simulink model "SM_Tq_Ctrl"  (R2023a)
settings: Solver=ode45  StartTime=0  StopTime=20  FixedStep=0.001  RelTol=1e-3  AbsTol=1e-6
libraries: simulink x11, dspsigops x4, Solver_SF x1
settings Model: ExtModeTrigMode=oneshot  Creator=jhu  LastModifiedBy=USER
settings SolverCC: AutoScaleAbsTol=off  AlgebraicLoopSolver=TrustRegion
settings DataIOCC: SaveFormat=Array  SignalLoggingSaveFormat=ModelDataLogs  ReturnWorkspaceOutputs=off  SignalLoggingName=sigsOut
settings OptimizationCC: BlockReduction=off  BooleanDataType=off  ExpressionDepthLimit=2147483647  LifeSpan=inf
settings DebuggingCC: SaveWithParameterizedLinksMsg=none  UnderspecifiedInitializationDetection=Classic  MergeDetectMultiDrivingBlocksExec=none  SignalResolutionControl=TryResolveAllWithWarning  MultiTaskDSMMsg=warning  MultiTaskCondExecSysMsg=none  FcnCallInpInsideContextMsg=warning  UnconnectedInputMsg=warning  UnconnectedOutputMsg=warning  UnconnectedLineMsg=warning  StateNameClashWarn=warning  SFUnexpectedBacktrackingDiag=warning  SFNoUnconditionalDefaultTransitionDiag=warning  SFExecutionAtInitializationDiag=none  ArithmeticOperatorsInVariantConditions=warning
settings HardwareCC: ProdBitPerPointer=32  ProdBitPerSizeT=32  ProdBitPerPtrDiffT=32  ProdLargestAtomicFloat=None  ProdIntDivRoundTo=Undefined  ProdEndianess=Unspecified  ProdWordSize=32  ProdHWDeviceType=32-bit Generic  TargetUnknown=on
settings ModelReferenceCC: PropagateSignalLabelsOutOfModel=off
settings SFSimCC: SimUseLocalCustomCode=off  CustomCodeUndefinedFunction=UseInterfaceOnly
settings RTWCC: TemplateMakefile=grt_vc.tmf  RTWUseLocalCustomCode=off
settings CodeAppCC: StateflowObjectComments=on
settings GRTTargetCC: TargetFcnLib=ansi_tfl_tmw.mat  TargetLangStandard=C89/C90 (ANSI)  CombineOutputUpdateFcns=off  GRTInterface=on
settings ConfigComp: CovMetricSettings=dw  CovSaveCumulativeToWorkspaceVar=on  CovSaveSingleToWorkspaceVar=on  CovExternalEMLEnable=off

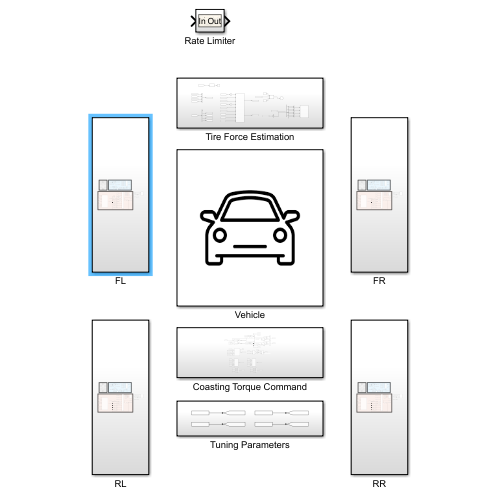
[thumbnail: Simulink's stored preview of the top-level diagram]
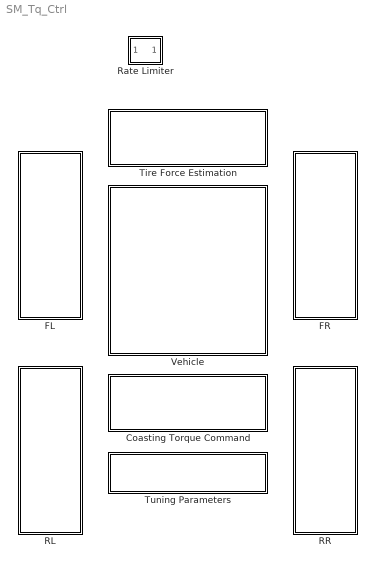
== system SM_Tq_Ctrl ==
  Coasting Torque Command : Subsystem
  FL : Subsystem
  FR : Subsystem
  RL : Subsystem
  RR : Subsystem
  Rate Limiter : Subsystem
  Tire Force Estimation : Subsystem
  Tuning Parameters : Subsystem
  Vehicle : Subsystem
      mask Display: image('C:\Users\USER\Downloads\vehicle_icon.png'); % Use "Edit Image" on toolstrip to change.

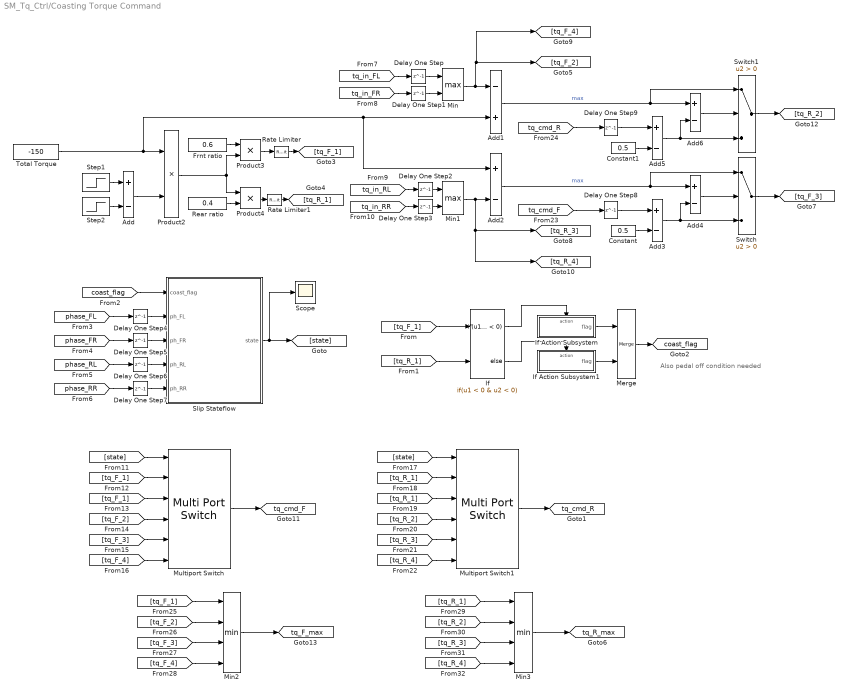
== system SM_Tq_Ctrl/Coasting Torque Command ==
  note: Also pedal off condition needed
  Add{,2..6} (6 alike) : Sum  Inputs=+-
  Add1 : Sum  Inputs=-+
  Constant : Constant  Value=0.5
  Constant1 : Constant  Value=0.5
  Delay One Step{,1..7} (8 alike) : Delay  DelayLength=1
  Delay One Step8 : Delay  DelayLength=1  SampleTime=0.01
  Delay One Step9 : Delay  DelayLength=1  SampleTime=0.01
  Frnt ratio : Constant  Value=0.6  SampleTime=0.01
  If : If  NumInputs=2  IfExpression=u1 < 0 & u2 < 0
  If Action Subsystem : Subsystem  TreatAsAtomicUnit=on
  If Action Subsystem1 : Subsystem  TreatAsAtomicUnit=on
  Merge : Merge
  Min : MinMax  Function=max  Inputs=2
  Min1 : MinMax  Function=max  Inputs=2
  Min2 : MinMax  Inputs=4
  Min3 : MinMax  Inputs=4
  Multiport Switch : MultiPortSwitch  DataPortOrder=Zero-based contiguous  Inputs=5  zeroidx=on  SaturateOnIntegerOverflow=off  InputSameDT=off
  Multiport Switch1 : MultiPortSwitch  DataPortOrder=Zero-based contiguous  Inputs=5  zeroidx=on  SaturateOnIntegerOverflow=off  InputSameDT=off
  Product2 : Product
  Product3 : Product
  Product4 : Product
  Rate Limiter : RateLimiter  RisingSlewLimit=600  FallingSlewLimit=-600  SampleTimeMode=inherited
  Rate Limiter1 : RateLimiter  RisingSlewLimit=600  FallingSlewLimit=-600  SampleTimeMode=inherited
  Rear ratio : Constant  Value=0.4  SampleTime=0.01
  Scope : Scope
  Slip Stateflow : Stateflow chart  TreatAsAtomicUnit=on
  Step1 : Step  Time=5  SampleTime=0.01
  Step2 : Step  Time=10  SampleTime=0.01
  Switch : Switch  Criteria=u2 > Threshold  SaturateOnIntegerOverflow=off  InputSameDT=off
  Switch1 : Switch  Criteria=u2 > Threshold  SaturateOnIntegerOverflow=off  InputSameDT=off
  Total Torque : Constant  Value=-150  VectorParams1D=off  SampleTime=0.01
  tag scope: coast_flag=global, tq_F_max=global, tq_R_max=global, tq_cmd_F=global, tq_cmd_R=global
  wires:
  [tq_F_1] -> If/1
  [tq_R_1] -> If/2
  If/1 -> If Action Subsystem/Action
  If Action Subsystem/1(flag) -> Merge/1
  If Action Subsystem1/1(flag) -> Merge/2
  If/2 -> If Action Subsystem1/Action
  Merge/1 -> [coast_flag]
  [coast_flag] -> Slip Stateflow/1(coast_flag)
  [phase_FL] -> Delay One Step4/1
  [phase_FR] -> Delay One Step5/1
  [phase_RL] -> Delay One Step6/1
  [phase_RR] -> Delay One Step7/1
  Slip Stateflow/1(state) -> Scope/1, [state]
  Step1/1 -> Add/1
  Step2/1 -> Add/2
  Add/1 -> Product2/2
  Product2/1 -> Product4/1, Product3/2
  Frnt ratio/1 -> Product3/1
  Rear ratio/1 -> Product4/2
  Product3/1 -> Rate Limiter/1
  Product4/1 -> Rate Limiter1/1
  [tq_in_FL] -> Delay One Step/1
  [tq_in_FR] -> Delay One Step1/1
  Min/1 -> [tq_F_4], [tq_F_2], Add1/1
  [tq_in_RL] -> Delay One Step2/1
  [tq_in_RR] -> Delay One Step3/1
  Min1/1 -> [tq_R_4], [tq_R_3], Add2/2
  Add2/1 -> Switch/1, Add4/1  "max"
  [state] -> Multiport Switch/1
  [tq_F_1] -> Multiport Switch/2
  [tq_F_1] -> Multiport Switch/3
  [tq_F_2] -> Multiport Switch/4
  [tq_F_3] -> Multiport Switch/5
  [tq_F_4] -> Multiport Switch/6
  Multiport Switch/1 -> [tq_cmd_F]
  Multiport Switch1/1 -> [tq_cmd_R]
  [tq_R_3] -> Multiport Switch1/5
  [tq_R_4] -> Multiport Switch1/6
  [tq_R_2] -> Multiport Switch1/4
  [tq_R_1] -> Multiport Switch1/2
  [state] -> Multiport Switch1/1
  [tq_R_1] -> Multiport Switch1/3
  Delay One Step/1 -> Min/1
  Delay One Step1/1 -> Min/2
  Delay One Step2/1 -> Min1/1
  Delay One Step3/1 -> Min1/2
  Delay One Step4/1 -> Slip Stateflow/2(ph_FL)
  Delay One Step5/1 -> Slip Stateflow/3(ph_FR)
  Delay One Step6/1 -> Slip Stateflow/4(ph_RL)
  Delay One Step7/1 -> Slip Stateflow/5(ph_RR)
  [tq_cmd_F] -> Delay One Step8/1
  Delay One Step8/1 -> Add3/1
  Constant/1 -> Add3/2
  Add3/1 -> Add4/2, Switch/3
  Add4/1 -> Switch/2
  Switch/1 -> [tq_F_3]
  Switch1/1 -> [tq_R_2]
  Delay One Step9/1 -> Add5/1
  Add1/1 -> Switch1/1, Add6/1  "max"
  Add6/1 -> Switch1/2
  [tq_cmd_R] -> Delay One Step9/1
  Add5/1 -> Add6/2, Switch1/3
  Constant1/1 -> Add5/2
  Min2/1 -> [tq_F_max]
  [tq_F_1] -> Min2/1
  [tq_F_2] -> Min2/2
  [tq_F_3] -> Min2/3
  [tq_F_4] -> Min2/4
  Min3/1 -> [tq_R_max]
  [tq_R_1] -> Min3/1
  [tq_R_2] -> Min3/2
  [tq_R_3] -> Min3/3
  [tq_R_4] -> Min3/4
  Total Torque/1 -> Add2/1, Add1/2, Product2/1
  Rate Limiter/1 -> [tq_F_1]
  Rate Limiter1/1 -> [tq_R_1]

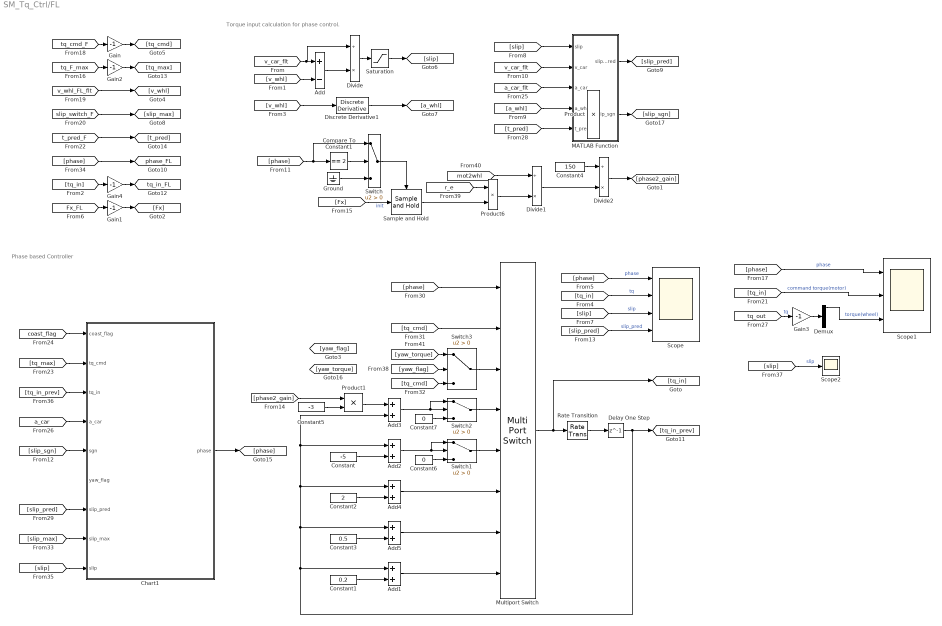
== system SM_Tq_Ctrl/FL ==
  note: Phase based Controller
  note: Torque input calculation for phase control.
  Add : Sum  Inputs=+-
  Add{1..5} (5 alike) : Sum
  Chart1 : Stateflow chart  TreatAsAtomicUnit=on
      settings: PortSchema="{\"entries\":[{\"content\":{\"sides\":[{\"content\":{\"connectorIds\":[\"In3\",\"In6\",\"In7\",\"In2\",\"In8\",\"In9\",\"In4\",\"In5\",\"In1\"]},\"type\":\"ConnectorPlacement.EquallySpacedRectSide\",\"uuid\":\"d1b40d47-5080-4bdb-9b64-2db0b8a6d570\"},{\"content\":{\"connectorIds\":[\"Out1\"],\"side\":\"RIGHT\"},\"type\":\"ConnectorPlacement.EquallySpacedRectSide\",\"uuid\":\"3562d231-244b-4945-a90c-51a654d62f0f\"},{\"content\":{\"side\":\"TOP\"},\"type\":\"ConnectorPlacement.EquallySpacedRectSide\",\"uuid\":\"6c914ffe-04dc-4ab2-bade-76d69248353c\"}]},\"type\":\"ConnectorPlacement.EquallySpacedConnector\",\"uuid\":\"36a59ec9-6bc3-461d-a020-c1da85e3b47f\"}],\"packageUris\":[\"http://schema.mathworks.com/mf0/Connector/R2020b\"],\"version\":\"1.0\"}"
  Compare To Constant1 : simulink/Logic and Bit Operations/Compare To Constant  relop===  const=2  OutDataTypeStr=boolean
  Constant : Constant  Value=-5
  Constant1 : Constant  Value=0.2
  Constant2 : Constant  Value=2
  Constant3 : Constant  Value=0.5
  Constant4 : Constant  Value=150
  Constant5 : Constant  Value=-3
  Constant6 : Constant  Value=0
  Constant7 : Constant  Value=0
  Delay One Step : Delay  DelayLength=1  SampleTime=0.01
  Demux : Demux
  Discrete Derivative1 : simulink/Discrete/Discrete Derivative  gainval=1.0  ICPrevScaledInput=0.0  OutMin=[]  OutMax=[]  OutDataType=fixdt(1, 16)  OutScaling=2^-10  DoSatur=off
  Divide : Product  Inputs=/*
  Divide1 : Product  Inputs=/*
  Divide2 : Product  Inputs=/*
  Gain{,1..4} (5 alike) : Gain  Gain=-1
  Ground : Ground
  MATLAB Function : MATLAB Function  TreatAsAtomicUnit=on
  Multiport Switch : MultiPortSwitch  DataPortOrder=Zero-based contiguous  Inputs=7  zeroidx=on  SaturateOnIntegerOverflow=off  InputSameDT=off
  Product : Product
  Product1 : Product
  Product6 : Product
  Rate Transition : RateTransition  OutPortSampleTime=0.01
  Sample and Hold : dspsigops/Sample and Hold  trig=Rising edge  initCond=0  latchinput=off
  Saturation : Saturate  UpperLimit=1  LowerLimit=-1
  Scope : Scope  NumInputPorts=4
  Scope1 : Scope  NumInputPorts=3
  Scope2 : Scope
  Switch{,1..3} (4 alike) : Switch  Criteria=u2 > Threshold  SaturateOnIntegerOverflow=off  InputSameDT=off
  tag scope: phase_FL=global, tq_in_FL=global
  wires:
  [v_car_flt] -> Divide/1, Add/1
  [v_whl] -> Add/2
  Add/1 -> Divide/2
  Divide/1 -> Saturation/1
  Saturation/1 -> [slip]
  [v_whl] -> Discrete Derivative1/1
  Discrete Derivative1/1 -> [a_whl]
  [slip_switch_F] -> [slip_max]
  [v_whl_FL_flt] -> [v_whl]
  [phase] -> Multiport Switch/1
  [tq_cmd] -> Multiport Switch/2
  [tq_cmd] -> Switch3/3
  Rate Transition/1 -> Delay One Step/1
  [slip] -> MATLAB Function/1(slip)
  [a_whl] -> MATLAB Function/4(a_whl)
  [v_car_flt] -> MATLAB Function/2(v_car)
  MATLAB Function/1(slip_pred) -> [slip_pred]
  [t_pred_F] -> [t_pred]
  [t_pred] -> MATLAB Function/5(t_pred)
  Add2/1 -> Switch1/1, Switch1/2
  Gain/1 -> [tq_cmd]
  Multiport Switch/1 -> [tq_in], Rate Transition/1
  Add4/1 -> Multiport Switch/6
  Constant2/1 -> Add4/2
  Constant3/1 -> Add5/2
  Add5/1 -> Multiport Switch/7
  Ground/1 -> Switch/3
  Switch/1 -> Sample and Hold/Trigger
  Sample and Hold/1 -> Product6/2
  [phase] -> Switch/1, Compare To Constant1/1
  Compare To Constant1/1 -> Switch/2
  Delay One Step/1 -> [tq_in_prev], Add3/2, Add2/1, Add4/1, Add5/1, Add1/1
  [Fx] -> Sample and Hold/1  "init"
  [tq_max] -> Chart1/6(tq_cmd)
  [coast_flag] -> Chart1/3(coast_flag)
  Chart1/1(phase) -> [phase]
  [a_car] -> Chart1/2(a_car)
  [slip_sgn] -> Chart1/8(sgn)
  [slip_pred] -> Chart1/4(slip_pred)
  [slip_max] -> Chart1/5(slip_max)
  [slip] -> Chart1/1(slip)
  [tq_in_prev] -> Chart1/7(tq_in)
  [phase] -> Scope/1  "phase"
  [tq_in] -> Scope/2  "tq"
  [slip] -> Scope/3  "slip"
  Divide1/1 -> Divide2/2
  [slip_pred] -> Scope/4  "slip_pred"
  Add3/1 -> Switch2/1, Switch2/2
  [phase] -> [phase_FL]
  [tq_cmd_F] -> Gain/1
  [tq_F_max] -> Gain2/1
  Gain2/1 -> [tq_max]
  [a_car_flt] -> MATLAB Function/3(a_car)
  [tq_in] -> Gain4/1
  Gain4/1 -> [tq_in_FL]
  [Fx_FL] -> Gain1/1
  Gain1/1 -> [Fx]
  [r_e] -> Product6/1
  Product6/1 -> Divide1/2
  [mot2whl] -> Divide1/1
  Constant/1 -> Add2/2
  Add1/1 -> Multiport Switch/8
  Constant1/1 -> Add1/2
  MATLAB Function/2(slip_sgn) -> [slip_sgn]
  [phase] -> Scope1/1  "phase"
  [tq_in] -> Scope1/2  "command torque(motor)"
  [tq_out] -> Gain3/1  "tq"
  Gain3/1 -> Demux/1
  Demux/1 -> Scope1/3  "torque(wheel)"
  [slip] -> Scope2/1  "slip"
  Divide2/1 -> [phase2_gain]
  Constant4/1 -> Divide2/1
  [phase2_gain] -> Product1/1
  Constant5/1 -> Product1/2
  Product1/1 -> Add3/1
  Switch1/1 -> Multiport Switch/5
  Constant6/1 -> Switch1/3
  Switch2/1 -> Multiport Switch/4
  Constant7/1 -> Switch2/3
  [yaw_flag] -> Switch3/2
  [yaw_torque] -> Switch3/1
  Switch3/1 -> Multiport Switch/3

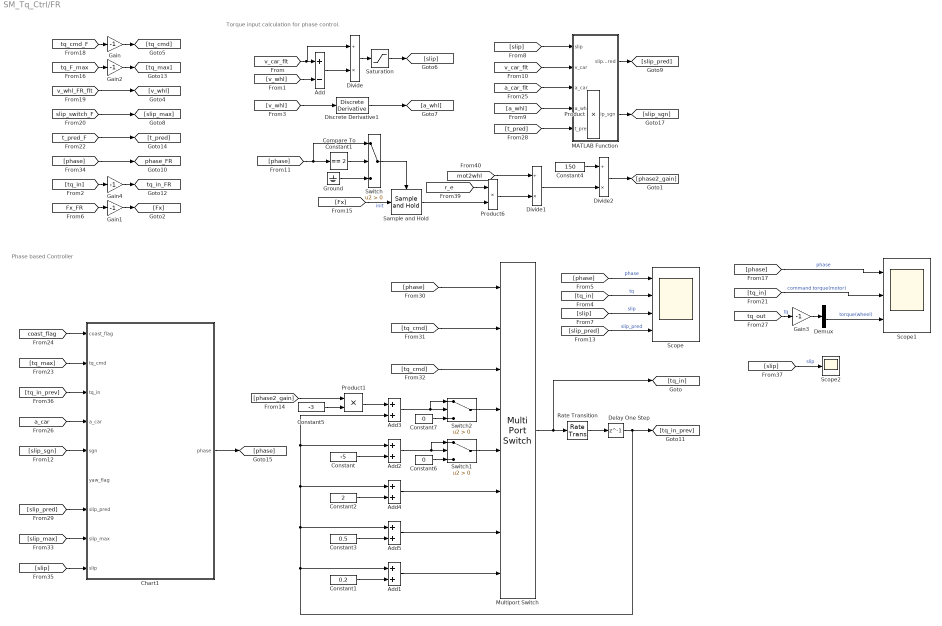
== system SM_Tq_Ctrl/FR ==
  note: Torque input calculation for phase control.
  note: Phase based Controller
  Add : Sum  Inputs=+-
  Add{1..5} (5 alike) : Sum
  Chart1 : Stateflow chart  TreatAsAtomicUnit=on
      settings: PortSchema="{\"entries\":[{\"content\":{\"sides\":[{\"content\":{\"connectorIds\":[\"In3\",\"In6\",\"In7\",\"In2\",\"In8\",\"In9\",\"In4\",\"In5\",\"In1\"]},\"type\":\"ConnectorPlacement.EquallySpacedRectSide\",\"uuid\":\"d1b40d47-5080-4bdb-9b64-2db0b8a6d570\"},{\"content\":{\"connectorIds\":[\"Out1\"],\"side\":\"RIGHT\"},\"type\":\"ConnectorPlacement.EquallySpacedRectSide\",\"uuid\":\"3562d231-244b-4945-a90c-51a654d62f0f\"},{\"content\":{\"side\":\"TOP\"},\"type\":\"ConnectorPlacement.EquallySpacedRectSide\",\"uuid\":\"6c914ffe-04dc-4ab2-bade-76d69248353c\"}]},\"type\":\"ConnectorPlacement.EquallySpacedConnector\",\"uuid\":\"36a59ec9-6bc3-461d-a020-c1da85e3b47f\"}],\"packageUris\":[\"http://schema.mathworks.com/mf0/Connector/R2020b\"],\"version\":\"1.0\"}"
  Compare To Constant1 : simulink/Logic and Bit Operations/Compare To Constant  relop===  const=2  OutDataTypeStr=boolean
  Constant : Constant  Value=-5
  Constant1 : Constant  Value=0.2
  Constant2 : Constant  Value=2
  Constant3 : Constant  Value=0.5
  Constant4 : Constant  Value=150
  Constant5 : Constant  Value=-3
  Constant6 : Constant  Value=0
  Constant7 : Constant  Value=0
  Delay One Step : Delay  DelayLength=1  SampleTime=0.01
  Demux : Demux
  Discrete Derivative1 : simulink/Discrete/Discrete Derivative  gainval=1.0  ICPrevScaledInput=0.0  OutMin=[]  OutMax=[]  OutDataType=fixdt(1, 16)  OutScaling=2^-10  DoSatur=off
  Divide : Product  Inputs=/*
  Divide1 : Product  Inputs=/*
  Divide2 : Product  Inputs=/*
  Gain{,1..4} (5 alike) : Gain  Gain=-1
  Ground : Ground
  MATLAB Function : MATLAB Function  TreatAsAtomicUnit=on
  Multiport Switch : MultiPortSwitch  DataPortOrder=Zero-based contiguous  Inputs=7  zeroidx=on  SaturateOnIntegerOverflow=off  InputSameDT=off
  Product : Product
  Product1 : Product
  Product6 : Product
  Rate Transition : RateTransition  OutPortSampleTime=0.01
  Sample and Hold : dspsigops/Sample and Hold  trig=Rising edge  initCond=0  latchinput=off
  Saturation : Saturate  UpperLimit=1  LowerLimit=-1
  Scope : Scope  NumInputPorts=4
  Scope1 : Scope  NumInputPorts=3
  Scope2 : Scope
  Switch : Switch  Criteria=u2 > Threshold  SaturateOnIntegerOverflow=off  InputSameDT=off
  Switch1 : Switch  Criteria=u2 > Threshold  SaturateOnIntegerOverflow=off  InputSameDT=off
  Switch2 : Switch  Criteria=u2 > Threshold  SaturateOnIntegerOverflow=off  InputSameDT=off
  tag scope: phase_FR=global, tq_in_FR=global
  wires:
  Constant7/1 -> Switch2/3
  Switch2/1 -> Multiport Switch/4
  Constant6/1 -> Switch1/3
  Switch1/1 -> Multiport Switch/5
  Product1/1 -> Add3/1
  Constant5/1 -> Product1/2
  [phase2_gain] -> Product1/1
  Constant4/1 -> Divide2/1
  Divide2/1 -> [phase2_gain]
  [slip] -> Scope2/1  "slip"
  Demux/3 -> Scope1/3  "torque(wheel)"
  Gain3/1 -> Demux/1
  [tq_out] -> Gain3/1  "tq"
  [tq_in] -> Scope1/2  "command torque(motor)"
  [phase] -> Scope1/1  "phase"
  MATLAB Function/2(slip_sgn) -> [slip_sgn]
  Constant1/1 -> Add1/2
  Add1/1 -> Multiport Switch/8
  Constant/1 -> Add2/2
  [mot2whl] -> Divide1/1
  Product6/1 -> Divide1/2
  [r_e] -> Product6/1
  Gain1/1 -> [Fx]
  [Fx_FR] -> Gain1/1
  Gain4/1 -> [tq_in_FR]
  [tq_in] -> Gain4/1
  [a_car_flt] -> MATLAB Function/3(a_car)
  Gain2/1 -> [tq_max]
  [tq_F_max] -> Gain2/1
  [tq_cmd_F] -> Gain/1
  [phase] -> [phase_FR]
  Add3/1 -> Switch2/2, Switch2/1
  [slip_pred] -> Scope/4  "slip_pred"
  Divide1/1 -> Divide2/2
  [slip] -> Scope/3  "slip"
  [tq_in] -> Scope/2  "tq"
  [phase] -> Scope/1  "phase"
  [tq_in_prev] -> Chart1/7(tq_in)
  [slip] -> Chart1/1(slip)
  [slip_max] -> Chart1/5(slip_max)
  [slip_pred] -> Chart1/4(slip_pred)
  [slip_sgn] -> Chart1/8(sgn)
  [a_car] -> Chart1/2(a_car)
  Chart1/1(phase) -> [phase]
  [coast_flag] -> Chart1/3(coast_flag)
  [tq_max] -> Chart1/6(tq_cmd)
  [Fx] -> Sample and Hold/1  "init"
  Delay One Step/1 -> Add1/1, Add5/1, Add4/1, Add2/1, Add3/2, [tq_in_prev]
  Compare To Constant1/1 -> Switch/2
  [phase] -> Compare To Constant1/1, Switch/1
  Sample and Hold/1 -> Product6/2
  Switch/1 -> Sample and Hold/Trigger
  Ground/1 -> Switch/3
  Add5/1 -> Multiport Switch/7
  Constant3/1 -> Add5/2
  Constant2/1 -> Add4/2
  Add4/1 -> Multiport Switch/6
  Multiport Switch/1 -> Rate Transition/1, [tq_in]
  Gain/1 -> [tq_cmd]
  Add2/1 -> Switch1/2, Switch1/1
  [t_pred] -> MATLAB Function/5(t_pred)
  [t_pred_F] -> [t_pred]
  MATLAB Function/1(slip_pred) -> [slip_pred]
  [v_car_flt] -> MATLAB Function/2(v_car)
  [a_whl] -> MATLAB Function/4(a_whl)
  [slip] -> MATLAB Function/1(slip)
  Rate Transition/1 -> Delay One Step/1
  [tq_cmd] -> Multiport Switch/3
  [tq_cmd] -> Multiport Switch/2
  [phase] -> Multiport Switch/1
  [v_whl_FR_flt] -> [v_whl]
  [slip_switch_F] -> [slip_max]
  Discrete Derivative1/1 -> [a_whl]
  [v_whl] -> Discrete Derivative1/1
  Saturation/1 -> [slip]
  Divide/1 -> Saturation/1
  Add/1 -> Divide/2
  [v_whl] -> Add/2
  [v_car_flt] -> Add/1, Divide/1

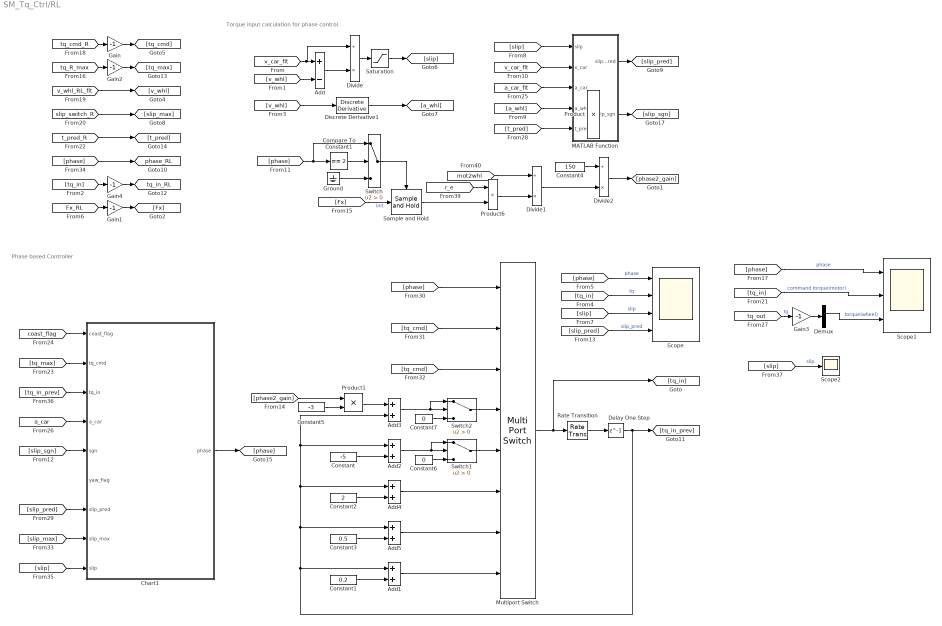
== system SM_Tq_Ctrl/RL ==
  note: Torque input calculation for phase control.
  note: Phase based Controller
  Add : Sum  Inputs=+-
  Add{1..5} (5 alike) : Sum
  Chart1 : Stateflow chart  TreatAsAtomicUnit=on
      settings: PortSchema="{\"entries\":[{\"content\":{\"sides\":[{\"content\":{\"connectorIds\":[\"In3\",\"In6\",\"In7\",\"In2\",\"In8\",\"In9\",\"In4\",\"In5\",\"In1\"]},\"type\":\"ConnectorPlacement.EquallySpacedRectSide\",\"uuid\":\"d1b40d47-5080-4bdb-9b64-2db0b8a6d570\"},{\"content\":{\"connectorIds\":[\"Out1\"],\"side\":\"RIGHT\"},\"type\":\"ConnectorPlacement.EquallySpacedRectSide\",\"uuid\":\"3562d231-244b-4945-a90c-51a654d62f0f\"},{\"content\":{\"side\":\"TOP\"},\"type\":\"ConnectorPlacement.EquallySpacedRectSide\",\"uuid\":\"6c914ffe-04dc-4ab2-bade-76d69248353c\"}]},\"type\":\"ConnectorPlacement.EquallySpacedConnector\",\"uuid\":\"36a59ec9-6bc3-461d-a020-c1da85e3b47f\"}],\"packageUris\":[\"http://schema.mathworks.com/mf0/Connector/R2020b\"],\"version\":\"1.0\"}"
  Compare To Constant1 : simulink/Logic and Bit Operations/Compare To Constant  relop===  const=2  OutDataTypeStr=boolean
  Constant : Constant  Value=-5
  Constant1 : Constant  Value=0.2
  Constant2 : Constant  Value=2
  Constant3 : Constant  Value=0.5
  Constant4 : Constant  Value=150
  Constant5 : Constant  Value=-3
  Constant6 : Constant  Value=0
  Constant7 : Constant  Value=0
  Delay One Step : Delay  DelayLength=1  SampleTime=0.01
  Demux : Demux
  Discrete Derivative1 : simulink/Discrete/Discrete Derivative  gainval=1.0  ICPrevScaledInput=0.0  OutMin=[]  OutMax=[]  OutDataType=fixdt(1, 16)  OutScaling=2^-10  DoSatur=off
  Divide : Product  Inputs=/*
  Divide1 : Product  Inputs=/*
  Divide2 : Product  Inputs=/*
  Gain{,1..4} (5 alike) : Gain  Gain=-1
  Ground : Ground
  MATLAB Function : MATLAB Function  TreatAsAtomicUnit=on
  Multiport Switch : MultiPortSwitch  DataPortOrder=Zero-based contiguous  Inputs=7  zeroidx=on  SaturateOnIntegerOverflow=off  InputSameDT=off
  Product : Product
  Product1 : Product
  Product6 : Product
  Rate Transition : RateTransition  OutPortSampleTime=0.01
  Sample and Hold : dspsigops/Sample and Hold  trig=Rising edge  initCond=0  latchinput=off
  Saturation : Saturate  UpperLimit=1  LowerLimit=-1
  Scope : Scope  NumInputPorts=4
  Scope1 : Scope  NumInputPorts=3
  Scope2 : Scope
  Switch : Switch  Criteria=u2 > Threshold  SaturateOnIntegerOverflow=off  InputSameDT=off
  Switch1 : Switch  Criteria=u2 > Threshold  SaturateOnIntegerOverflow=off  InputSameDT=off
  Switch2 : Switch  Criteria=u2 > Threshold  SaturateOnIntegerOverflow=off  InputSameDT=off
  tag scope: phase_RL=global, tq_in_RL=global
  wires:
  Constant7/1 -> Switch2/3
  Switch2/1 -> Multiport Switch/4
  Constant6/1 -> Switch1/3
  Switch1/1 -> Multiport Switch/5
  Product1/1 -> Add3/1
  Constant5/1 -> Product1/2
  [phase2_gain] -> Product1/1
  Constant4/1 -> Divide2/1
  Divide2/1 -> [phase2_gain]
  [slip] -> Scope2/1  "slip"
  Demux/2 -> Scope1/3  "torque(wheel)"
  Gain3/1 -> Demux/1
  [tq_out] -> Gain3/1  "tq"
  [tq_in] -> Scope1/2  "command torque(motor)"
  [phase] -> Scope1/1  "phase"
  MATLAB Function/2(slip_sgn) -> [slip_sgn]
  Constant1/1 -> Add1/2
  Add1/1 -> Multiport Switch/8
  Constant/1 -> Add2/2
  [mot2whl] -> Divide1/1
  Product6/1 -> Divide1/2
  [r_e] -> Product6/1
  Gain1/1 -> [Fx]
  [Fx_RL] -> Gain1/1
  Gain4/1 -> [tq_in_RL]
  [tq_in] -> Gain4/1
  [a_car_flt] -> MATLAB Function/3(a_car)
  Gain2/1 -> [tq_max]
  [tq_R_max] -> Gain2/1
  [tq_cmd_R] -> Gain/1
  [phase] -> [phase_RL]
  Add3/1 -> Switch2/2, Switch2/1
  [slip_pred] -> Scope/4  "slip_pred"
  Divide1/1 -> Divide2/2
  [slip] -> Scope/3  "slip"
  [tq_in] -> Scope/2  "tq"
  [phase] -> Scope/1  "phase"
  [tq_in_prev] -> Chart1/7(tq_in)
  [slip] -> Chart1/1(slip)
  [slip_max] -> Chart1/5(slip_max)
  [slip_pred] -> Chart1/4(slip_pred)
  [slip_sgn] -> Chart1/8(sgn)
  [a_car] -> Chart1/2(a_car)
  Chart1/1(phase) -> [phase]
  [coast_flag] -> Chart1/3(coast_flag)
  [tq_max] -> Chart1/6(tq_cmd)
  [Fx] -> Sample and Hold/1  "init"
  Delay One Step/1 -> Add1/1, Add5/1, Add4/1, Add2/1, Add3/2, [tq_in_prev]
  Compare To Constant1/1 -> Switch/2
  [phase] -> Compare To Constant1/1, Switch/1
  Sample and Hold/1 -> Product6/2
  Switch/1 -> Sample and Hold/Trigger
  Ground/1 -> Switch/3
  Add5/1 -> Multiport Switch/7
  Constant3/1 -> Add5/2
  Constant2/1 -> Add4/2
  Add4/1 -> Multiport Switch/6
  Multiport Switch/1 -> Rate Transition/1, [tq_in]
  Gain/1 -> [tq_cmd]
  Add2/1 -> Switch1/2, Switch1/1
  [t_pred] -> MATLAB Function/5(t_pred)
  [t_pred_R] -> [t_pred]
  MATLAB Function/1(slip_pred) -> [slip_pred]
  [v_car_flt] -> MATLAB Function/2(v_car)
  [a_whl] -> MATLAB Function/4(a_whl)
  [slip] -> MATLAB Function/1(slip)
  Rate Transition/1 -> Delay One Step/1
  [tq_cmd] -> Multiport Switch/3
  [tq_cmd] -> Multiport Switch/2
  [phase] -> Multiport Switch/1
  [v_whl_RL_flt] -> [v_whl]
  [slip_switch_R] -> [slip_max]
  Discrete Derivative1/1 -> [a_whl]
  [v_whl] -> Discrete Derivative1/1
  Saturation/1 -> [slip]
  Divide/1 -> Saturation/1
  Add/1 -> Divide/2
  [v_whl] -> Add/2
  [v_car_flt] -> Add/1, Divide/1

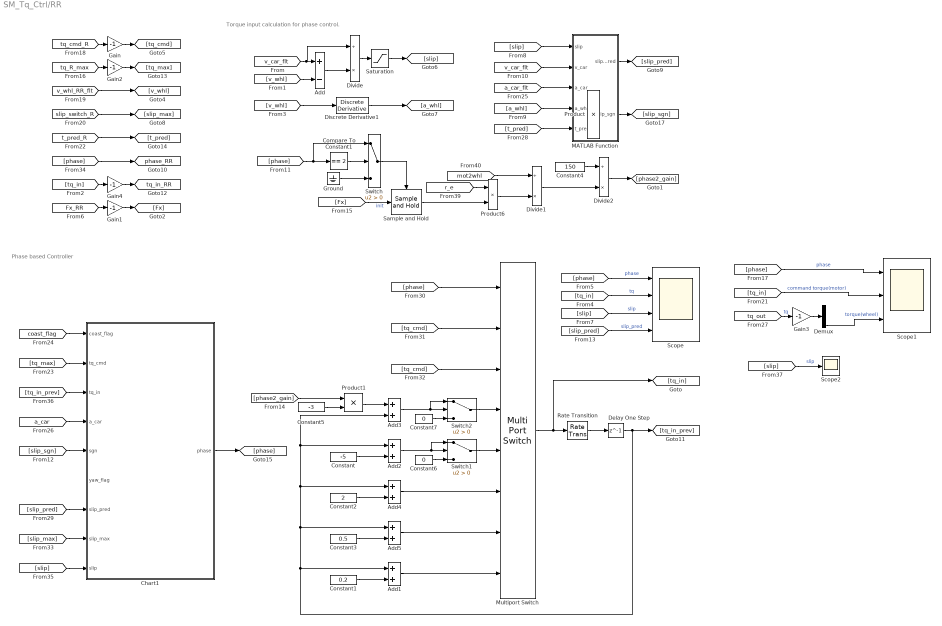
== system SM_Tq_Ctrl/RR ==
  note: Phase based Controller
  note: Torque input calculation for phase control.
  Add : Sum  Inputs=+-
  Add{1..5} (5 alike) : Sum
  Chart1 : Stateflow chart  TreatAsAtomicUnit=on
      settings: PortSchema="{\"entries\":[{\"content\":{\"sides\":[{\"content\":{\"connectorIds\":[\"In3\",\"In6\",\"In7\",\"In2\",\"In8\",\"In9\",\"In4\",\"In5\",\"In1\"]},\"type\":\"ConnectorPlacement.EquallySpacedRectSide\",\"uuid\":\"d1b40d47-5080-4bdb-9b64-2db0b8a6d570\"},{\"content\":{\"connectorIds\":[\"Out1\"],\"side\":\"RIGHT\"},\"type\":\"ConnectorPlacement.EquallySpacedRectSide\",\"uuid\":\"3562d231-244b-4945-a90c-51a654d62f0f\"},{\"content\":{\"side\":\"TOP\"},\"type\":\"ConnectorPlacement.EquallySpacedRectSide\",\"uuid\":\"6c914ffe-04dc-4ab2-bade-76d69248353c\"}]},\"type\":\"ConnectorPlacement.EquallySpacedConnector\",\"uuid\":\"36a59ec9-6bc3-461d-a020-c1da85e3b47f\"}],\"packageUris\":[\"http://schema.mathworks.com/mf0/Connector/R2020b\"],\"version\":\"1.0\"}"
  Compare To Constant1 : simulink/Logic and Bit Operations/Compare To Constant  relop===  const=2  OutDataTypeStr=boolean
  Constant : Constant  Value=-5
  Constant1 : Constant  Value=0.2
  Constant2 : Constant  Value=2
  Constant3 : Constant  Value=0.5
  Constant4 : Constant  Value=150
  Constant5 : Constant  Value=-3
  Constant6 : Constant  Value=0
  Constant7 : Constant  Value=0
  Delay One Step : Delay  DelayLength=1  SampleTime=0.01
  Demux : Demux
  Discrete Derivative1 : simulink/Discrete/Discrete Derivative  gainval=1.0  ICPrevScaledInput=0.0  OutMin=[]  OutMax=[]  OutDataType=fixdt(1, 16)  OutScaling=2^-10  DoSatur=off
  Divide : Product  Inputs=/*
  Divide1 : Product  Inputs=/*
  Divide2 : Product  Inputs=/*
  Gain{,1..4} (5 alike) : Gain  Gain=-1
  Ground : Ground
  MATLAB Function : MATLAB Function  TreatAsAtomicUnit=on
  Multiport Switch : MultiPortSwitch  DataPortOrder=Zero-based contiguous  Inputs=7  zeroidx=on  SaturateOnIntegerOverflow=off  InputSameDT=off
  Product : Product
  Product1 : Product
  Product6 : Product
  Rate Transition : RateTransition  OutPortSampleTime=0.01
  Sample and Hold : dspsigops/Sample and Hold  trig=Rising edge  initCond=0  latchinput=off
  Saturation : Saturate  UpperLimit=1  LowerLimit=-1
  Scope : Scope  NumInputPorts=4
  Scope1 : Scope  NumInputPorts=3
  Scope2 : Scope
  Switch : Switch  Criteria=u2 > Threshold  SaturateOnIntegerOverflow=off  InputSameDT=off
  Switch1 : Switch  Criteria=u2 > Threshold  SaturateOnIntegerOverflow=off  InputSameDT=off
  Switch2 : Switch  Criteria=u2 > Threshold  SaturateOnIntegerOverflow=off  InputSameDT=off
  tag scope: phase_RR=global, tq_in_RR=global
  wires:
  [v_car_flt] -> Divide/1, Add/1
  [v_whl] -> Add/2
  Add/1 -> Divide/2
  Divide/1 -> Saturation/1
  Saturation/1 -> [slip]
  [v_whl] -> Discrete Derivative1/1
  Discrete Derivative1/1 -> [a_whl]
  [slip_switch_R] -> [slip_max]
  [v_whl_RR_flt] -> [v_whl]
  [phase] -> Multiport Switch/1
  [tq_cmd] -> Multiport Switch/2
  [tq_cmd] -> Multiport Switch/3
  Rate Transition/1 -> Delay One Step/1
  [slip] -> MATLAB Function/1(slip)
  [a_whl] -> MATLAB Function/4(a_whl)
  [v_car_flt] -> MATLAB Function/2(v_car)
  MATLAB Function/1(slip_pred) -> [slip_pred]
  [t_pred_R] -> [t_pred]
  [t_pred] -> MATLAB Function/5(t_pred)
  Add2/1 -> Switch1/1, Switch1/2
  Gain/1 -> [tq_cmd]
  Multiport Switch/1 -> [tq_in], Rate Transition/1
  Add4/1 -> Multiport Switch/6
  Constant2/1 -> Add4/2
  Constant3/1 -> Add5/2
  Add5/1 -> Multiport Switch/7
  Ground/1 -> Switch/3
  Switch/1 -> Sample and Hold/Trigger
  Sample and Hold/1 -> Product6/2
  [phase] -> Switch/1, Compare To Constant1/1
  Compare To Constant1/1 -> Switch/2
  Delay One Step/1 -> [tq_in_prev], Add3/2, Add2/1, Add4/1, Add5/1, Add1/1
  [Fx] -> Sample and Hold/1  "init"
  [tq_max] -> Chart1/6(tq_cmd)
  [coast_flag] -> Chart1/3(coast_flag)
  Chart1/1(phase) -> [phase]
  [a_car] -> Chart1/2(a_car)
  [slip_sgn] -> Chart1/8(sgn)
  [slip_pred] -> Chart1/4(slip_pred)
  [slip_max] -> Chart1/5(slip_max)
  [slip] -> Chart1/1(slip)
  [tq_in_prev] -> Chart1/7(tq_in)
  [phase] -> Scope/1  "phase"
  [tq_in] -> Scope/2  "tq"
  [slip] -> Scope/3  "slip"
  Divide1/1 -> Divide2/2
  [slip_pred] -> Scope/4  "slip_pred"
  Add3/1 -> Switch2/1, Switch2/2
  [phase] -> [phase_RR]
  [tq_cmd_R] -> Gain/1
  [tq_R_max] -> Gain2/1
  Gain2/1 -> [tq_max]
  [a_car_flt] -> MATLAB Function/3(a_car)
  [tq_in] -> Gain4/1
  Gain4/1 -> [tq_in_RR]
  [Fx_RR] -> Gain1/1
  Gain1/1 -> [Fx]
  [r_e] -> Product6/1
  Product6/1 -> Divide1/2
  [mot2whl] -> Divide1/1
  Constant/1 -> Add2/2
  Add1/1 -> Multiport Switch/8
  Constant1/1 -> Add1/2
  MATLAB Function/2(slip_sgn) -> [slip_sgn]
  [phase] -> Scope1/1  "phase"
  [tq_in] -> Scope1/2  "command torque(motor)"
  [tq_out] -> Gain3/1  "tq"
  Gain3/1 -> Demux/1
  Demux/4 -> Scope1/3  "torque(wheel)"
  [slip] -> Scope2/1  "slip"
  Divide2/1 -> [phase2_gain]
  Constant4/1 -> Divide2/1
  [phase2_gain] -> Product1/1
  Constant5/1 -> Product1/2
  Product1/1 -> Add3/1
  Switch1/1 -> Multiport Switch/5
  Constant6/1 -> Switch1/3
  Switch2/1 -> Multiport Switch/4
  Constant7/1 -> Switch2/3

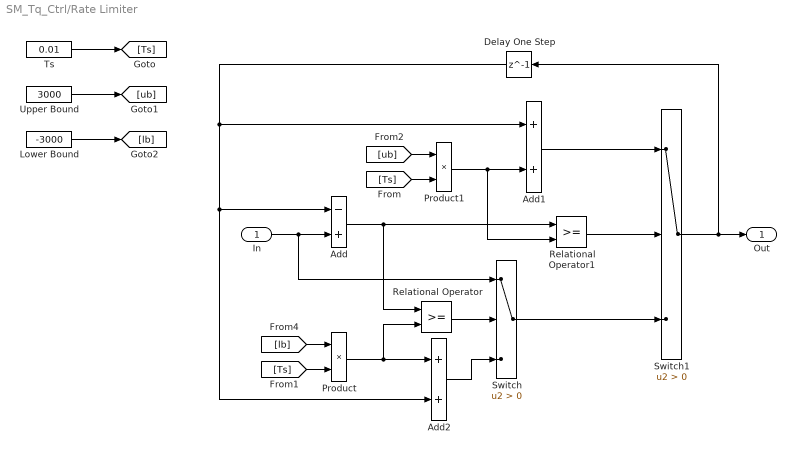
== system SM_Tq_Ctrl/Rate Limiter ==
  In : Inport
  Add : Sum  Inputs=-+
  Add1 : Sum
  Add2 : Sum
  Delay One Step : Delay  DelayLength=1  SampleTime=0.01
  Lower Bound : Constant  Value=-3000
  Product : Product
  Product1 : Product
  Relational Operator : RelationalOperator  OutDataTypeStr=boolean  RndMeth=Simplest  InputSameDT=off
  Relational Operator1 : RelationalOperator  OutDataTypeStr=boolean  RndMeth=Simplest  InputSameDT=off
  Switch : Switch  Criteria=u2 > Threshold  SaturateOnIntegerOverflow=off  InputSameDT=off
  Switch1 : Switch  Criteria=u2 > Threshold  SaturateOnIntegerOverflow=off  InputSameDT=off
  Ts : Constant  Value=0.01
  Upper Bound : Constant  Value=3000
  Out : Outport
  wires:
  In/1 -> Switch/1, Add/2
  Add/1 -> Relational Operator1/1, Relational Operator/1
  Relational Operator/1 -> Switch/2
  Product/1 -> Add2/1, Relational Operator/2
  Ts/1 -> [Ts]
  [Ts] -> Product1/2
  [Ts] -> Product/2
  Upper Bound/1 -> [ub]
  Lower Bound/1 -> [lb]
  [ub] -> Product1/1
  [lb] -> Product/1
  Product1/1 -> Relational Operator1/2, Add1/2
  Relational Operator1/1 -> Switch1/2
  Add1/1 -> Switch1/1
  Switch/1 -> Switch1/3
  Switch1/1 -> Delay One Step/1, Out/1
  Delay One Step/1 -> Add1/1, Add2/2, Add/1
  Add2/1 -> Switch/3

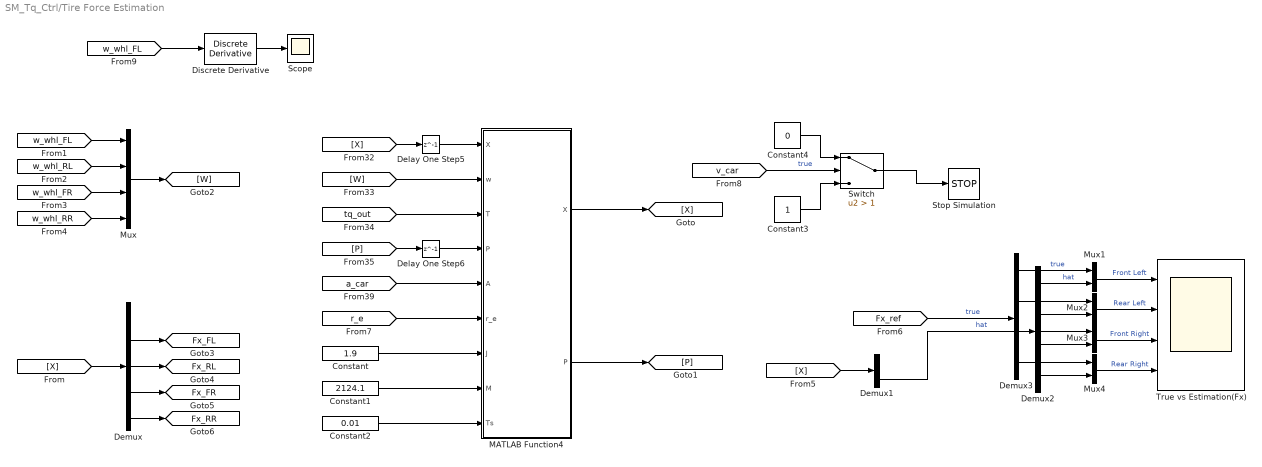
== system SM_Tq_Ctrl/Tire Force Estimation ==
  Constant : Constant  Value=1.9
  Constant1 : Constant  Value=2124.1
  Constant2 : Constant  Value=0.01
  Constant3 : Constant
  Constant4 : Constant  Value=0
  Delay One Step5 : Delay  DelayLength=1  InitialCondition=[64.1 64.1 64.1 64.1 0 0 0 0]'  SampleTime=0.01
  Delay One Step6 : Delay  DelayLength=1  InitialCondition=diag([64.1 64.1 64.1 64.1 0 0 0 0])  SampleTime=0.01
  Demux : Demux  Outputs=[4 1 1 1 1]
  Demux1 : Demux  Outputs=[4 4]
  Demux2 : Demux
  Demux3 : Demux
  Discrete Derivative : simulink/Discrete/Discrete Derivative  gainval=1.0  ICPrevScaledInput=0.0  OutMin=[]  OutMax=[]  OutDataType=fixdt(1, 16)  OutScaling=2^-10  DoSatur=off
  MATLAB Function4 : MATLAB Function  TreatAsAtomicUnit=on
  Mux : Mux
  Mux{1..4} (4 alike) : Mux  Inputs=2
  Scope : Scope
  Stop Simulation : Stop
  Switch : Switch  Criteria=u2 > Threshold  Threshold=1  SaturateOnIntegerOverflow=off  InputSameDT=off
  True vs Estimation(Fx) : Scope  NumInputPorts=4
  tag scope: Fx_FL=global, Fx_FR=global, Fx_RL=global, Fx_RR=global
  wires:
  [W] -> MATLAB Function4/2(w)
  [a_car] -> MATLAB Function4/5(A)
  [tq_out] -> MATLAB Function4/3(T)
  [P] -> Delay One Step6/1
  [X] -> Delay One Step5/1
  MATLAB Function4/1(X) -> [X]
  MATLAB Function4/2(P) -> [P]
  Delay One Step6/1 -> MATLAB Function4/4("P ")
  [w_whl_FL] -> Mux/1
  [w_whl_RL] -> Mux/2
  [w_whl_FR] -> Mux/3
  [w_whl_RR] -> Mux/4
  Mux/1 -> [W]
  Delay One Step5/1 -> MATLAB Function4/1("X ")
  [X] -> Demux/1
  Demux/2 -> [Fx_FL]
  [r_e] -> MATLAB Function4/6(r_e)
  Constant/1 -> MATLAB Function4/7(J)
  Constant2/1 -> MATLAB Function4/9(Ts)
  Constant1/1 -> MATLAB Function4/8(M)
  Demux/5 -> [Fx_RR]
  Demux/4 -> [Fx_FR]
  Demux/3 -> [Fx_RL]
  [X] -> Demux1/1
  Mux2/1 -> True vs Estimation(Fx)/2  "Rear Left"
  Demux3/3 -> Mux3/1
  Mux4/1 -> True vs Estimation(Fx)/4  "Rear Right"
  Demux3/1 -> Mux1/1  "true"
  Demux3/4 -> Mux4/1
  Demux2/1 -> Mux1/2  "hat"
  Demux2/4 -> Mux4/2
  Demux1/2 -> Demux2/1  "hat"
  [Fx_ref] -> Demux3/1  "true"
  Demux3/2 -> Mux2/1
  Mux3/1 -> True vs Estimation(Fx)/3  "Front Right"
  Demux2/2 -> Mux2/2
  Demux2/3 -> Mux3/2
  Mux1/1 -> True vs Estimation(Fx)/1  "Front Left"
  Constant3/1 -> Switch/3
  Switch/1 -> Stop Simulation/1
  Constant4/1 -> Switch/1
  [v_car] -> Switch/2  "true"
  [w_whl_FL] -> Discrete Derivative/1
  Discrete Derivative/1 -> Scope/1

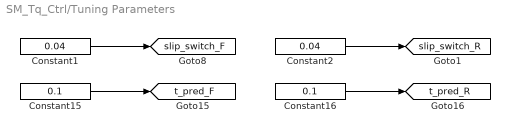
== system SM_Tq_Ctrl/Tuning Parameters ==
  Constant1 : Constant  Value=0.04  SampleTime=0.01
  Constant15 : Constant  Value=0.1  SampleTime=0.01
  Constant16 : Constant  Value=0.1  SampleTime=0.01
  Constant2 : Constant  Value=0.04  SampleTime=0.01
  tag scope: slip_switch_F=global, slip_switch_R=global, t_pred_F=global, t_pred_R=global
  wires:
  Constant1/1 -> [slip_switch_F]
  Constant2/1 -> [slip_switch_R]
  Constant15/1 -> [t_pred_F]
  Constant16/1 -> [t_pred_R]

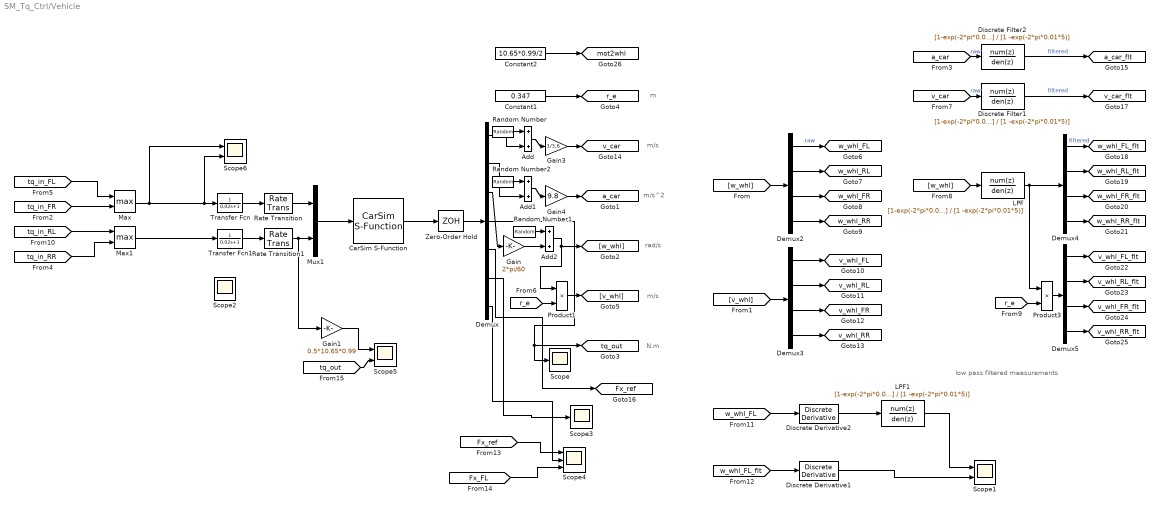
== system SM_Tq_Ctrl/Vehicle ==
  note: low pass filtered measurements
  note: m/s
  note: m
  note: m/s
  note: rad/s
  note: N.m
  note: m/s^2
  Add : Sum
  Add1 : Sum
  Add2 : Sum
  CarSim S-Function : Solver_SF/CarSim S-Function  Priority=1  SIMFILE=simfile.sim  Run_RTs=off  vs_state_ind=Run  StopMode_ind=Vehicle Model
  Constant1 : Constant  Value=0.347
  Constant2 : Constant  Value=10.65*0.99/2
  Demux : Demux  Outputs=[1 1 4 4 4 4 4]
  Demux{2..5} (4 alike) : Demux
  Discrete Derivative1 : simulink/Discrete/Discrete Derivative  gainval=1.0  ICPrevScaledInput=0.0  OutMin=[]  OutMax=[]  OutDataType=fixdt(1, 16)  OutScaling=2^-10  DoSatur=off
  Discrete Derivative2 : simulink/Discrete/Discrete Derivative  gainval=1.0  ICPrevScaledInput=0.0  OutMin=[]  OutMax=[]  OutDataType=fixdt(1, 16)  OutScaling=2^-10  DoSatur=off
  Discrete Filter1 : DiscreteFilter  Numerator=[1-exp(-2*pi*0.01*5)]  Denominator=[1 -exp(-2*pi*0.01*5)]  InitialStates=19.45  SampleTime=0.01
  Discrete Filter2 : DiscreteFilter  Numerator=[1-exp(-2*pi*0.01*5)]  Denominator=[1 -exp(-2*pi*0.01*5)]  SampleTime=0.01
  Gain : Gain  Gain=2*pi/60
  Gain1 : Gain  Gain=0.5*10.65*0.99
  Gain3 : Gain  Gain=1/3.6
  Gain4 : Gain  Gain=9.8
  LPF : DiscreteFilter  Numerator=[1-exp(-2*pi*0.01*5)]  Denominator=[1 -exp(-2*pi*0.01*5)]  InitialStates=56  SampleTime=0.01
  LPF1 : DiscreteFilter  Numerator=[1-exp(-2*pi*0.01*5)]  Denominator=[1 -exp(-2*pi*0.01*5)]  SampleTime=0.01
  Max : MinMax  Function=max  Inputs=2
  Max1 : MinMax  Function=max  Inputs=2
  Mux1 : Mux  Inputs=2
  Product1 : Product
  Product3 : Product
  Random Number : RandomNumber  Variance=0.0005  Seed=2  SampleTime=0.01
  Random Number1 : RandomNumber  Variance=0.002  Seed=2  SampleTime=0.01
  Random Number2 : RandomNumber  Variance=0.0002  Seed=2  SampleTime=0.01
  Rate Transition : RateTransition  OutPortSampleTime=0.01
  Rate Transition1 : RateTransition  OutPortSampleTime=0.01
  Scope : Scope
  Scope1 : Scope  NumInputPorts=2
  Scope2 : Scope
  Scope3 : Scope
  Scope4 : Scope  NumInputPorts=3
  Scope5 : Scope  NumInputPorts=2
  Scope6 : Scope  NumInputPorts=2
  Transfer Fcn : TransferFcn  Denominator=[0.02 1]
  Transfer Fcn1 : TransferFcn  Denominator=[0.02 1]
  Zero-Order Hold : ZeroOrderHold  SampleTime=0.01
  tag scope: Fx_ref=global, a_car=global, a_car_flt=global, mot2whl=global, r_e=global, tq_out=global, v_car=global, v_car_flt=global, v_whl_FL=global, v_whl_FL_flt=global, v_whl_FR=global, v_whl_FR_flt=global, v_whl_RL=global, v_whl_RL_flt=global, v_whl_RR=global, v_whl_RR_flt=global, w_whl_FL=global, w_whl_FL_flt=global, w_whl_FR=global, w_whl_FR_flt=global, w_whl_RL=global, w_whl_RL_flt=global, w_whl_RR=global, w_whl_RR_flt=global
  wires:
  Constant1/1 -> [r_e]
  [r_e] -> Product1/2
  Product1/1 -> [v_whl]
  Demux3/4 -> [v_whl_RR]
  Demux3/2 -> [v_whl_RL]
  [v_whl] -> Demux3/1
  Demux3/1 -> [v_whl_FL]
  Demux3/3 -> [v_whl_FR]
  Gain/1 -> Add2/2
  Demux/2 -> Add1/2
  Demux/3 -> Gain/1
  Gain4/1 -> [a_car]
  Demux/4 -> Scope/1, [tq_out]
  CarSim S-Function/1 -> Zero-Order Hold/1
  Demux2/2 -> [w_whl_RL]
  Gain3/1 -> [v_car]
  Demux2/1 -> [w_whl_FL]  "raw"
  Demux/1 -> Add/2
  Demux2/3 -> [w_whl_FR]
  Zero-Order Hold/1 -> Demux/1
  [w_whl] -> Demux2/1
  Demux2/4 -> [w_whl_RR]
  Transfer Fcn/1 -> Rate Transition/1
  Transfer Fcn1/1 -> Rate Transition1/1
  Mux1/1 -> CarSim S-Function/1
  Rate Transition/1 -> Mux1/1
  Rate Transition1/1 -> Gain1/1, Mux1/2
  [tq_in_FR] -> Max/2
  Random Number/1 -> Add/1
  Add/1 -> Gain3/1
  Random Number2/1 -> Add1/1
  Add1/1 -> Gain4/1
  Random Number1/1 -> Add2/1
  Add2/1 -> Product1/1, [w_whl]
  [v_car] -> Discrete Filter1/1  "raw"
  Discrete Filter1/1 -> [v_car_flt]  "filtered"
  [w_whl] -> LPF/1
  LPF/1 -> Demux4/1, Product3/1
  Demux4/1 -> [w_whl_FL_flt]  "filtered"
  Demux4/2 -> [w_whl_RL_flt]
  Demux4/3 -> [w_whl_FR_flt]
  Demux4/4 -> [w_whl_RR_flt]
  [r_e] -> Product3/2
  Product3/1 -> Demux5/1
  Demux5/1 -> [v_whl_FL_flt]
  Demux5/2 -> [v_whl_RL_flt]
  Demux5/3 -> [v_whl_FR_flt]
  Demux5/4 -> [v_whl_RR_flt]
  [a_car] -> Discrete Filter2/1  "raw"
  Discrete Filter2/1 -> [a_car_flt]  "filtered"
  [tq_in_FL] -> Max/1
  [tq_in_RR] -> Max1/2
  [tq_in_RL] -> Max1/1
  [w_whl_FL_flt] -> Discrete Derivative1/1
  Discrete Derivative1/1 -> Scope1/2
  [w_whl_FL] -> Discrete Derivative2/1
  Discrete Derivative2/1 -> LPF1/1
  LPF1/1 -> Scope1/1
  Demux/5 -> [Fx_ref]
  Demux/6 -> Scope3/1
  Demux/7 -> Scope4/2
  [Fx_ref] -> Scope4/1
  [Fx_FL] -> Scope4/3
  [tq_out] -> Scope5/2
  Gain1/1 -> Scope5/1
  Constant2/1 -> [mot2whl]
  Max/1 -> Scope6/2, Transfer Fcn/1, Scope6/1
  Max1/1 -> Transfer Fcn1/1

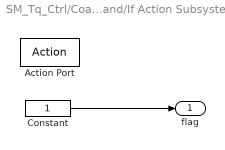
== system SM_Tq_Ctrl/Coasting Torque Command/If Action Subsystem ==
  Action Port : ActionPort  ActionPortLabel=if(u1 < 0 & u2 < 0)
  Constant : Constant  SampleTime=0.01
  flag : Outport
  wires:
  Constant/1 -> flag/1

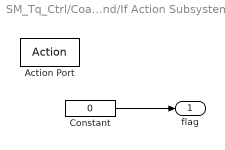
== system SM_Tq_Ctrl/Coasting Torque Command/If Action Subsystem1 ==
  Action Port : ActionPort  ActionPortLabel=else
  Constant : Constant  Value=0  SampleTime=0.01
  flag : Outport
  wires:
  Constant/1 -> flag/1

== stateflow chart SM_Tq_Ctrl/RR/Chart1 ==
  state LSC_On
    state Phase6
      entry,during:
      phase = 6;
    state Phase1
      entry,during:
      phase = 1;
    state Phase2
      entry,during:
      phase = 2;
    state Phase3
      entry,during:
      phase = 3;
    state Phase4
      entry,during:
      phase = 4;
    state Phase5
      entry,during:
      phase = 5;
    Phase6 -> (junction 225) [order 1] : [(yaw_flag == 1)]
    Phase6 -> (junction 235) [order 2] : [(slip > 0.85*slip_max)]
    (junction 225) -> Phase1
    (junction 235) -> (junction 167)
    Phase2 -> Phase6 [order 1] : [(slip_pred < 0.8*slip_max)]
    (default) -> Phase1
    Phase1 -> Phase2 : [(slip_pred > 0.95*slip_max)]
    (junction 167) -> Phase2
    (junction 165) -> (junction 167)
    (junction 217) -> Phase1
    Phase2 -> Phase3 [order 2] : [(slip > 0.9*slip_max)]
    Phase3 -> Phase4 : [(slip < 0.9*slip_max)]
    Phase4 -> (junction 217) [order 1] : [(tq_cmd < tq_in)]
    (junction 220) -> (junction 217)
    Phase4 -> Phase5 [order 2] : [(sgn > 0)]
    Phase5 -> (junction 220) [order 1] : [(tq_cmd < tq_in)]
    Phase5 -> (junction 165) [order 2] : [(slip_pred > 0.9*slip_max)]
  state LSC_off
    entry,during:
    phase = 0;
  state ready
    phase = 0;
  LSC_On -> (junction 231) : [(coast_flag ~= 1)]
  (junction 231) -> ready
  (default) -> ready
  LSC_off -> LSC_On : [(sgn > 0)&&(slip > 0)&&(a_car < 0)]
  ready -> LSC_off : [(coast_flag == 1)]
  data: phase output; slip input; a_car input; coast_flag input; slip_pred input; slip_max input; tq_cmd input; tq_in input; sgn input; yaw_flag input

== stateflow chart SM_Tq_Ctrl/RL/Chart1 ==
  state LSC_On
    state Phase6
      entry,during:
      phase = 6;
    state Phase1
      entry,during:
      phase = 1;
    state Phase2
      entry,during:
      phase = 2;
    state Phase3
      entry,during:
      phase = 3;
    state Phase4
      entry,during:
      phase = 4;
    state Phase5
      entry,during:
      phase = 5;
    Phase6 -> (junction 225) [order 1] : [(yaw_flag == 1)]
    Phase6 -> (junction 235) [order 2] : [(slip > 0.85*slip_max)]
    (junction 225) -> Phase1
    (junction 235) -> (junction 167)
    Phase2 -> Phase6 [order 1] : [(slip_pred < 0.8*slip_max)]
    (default) -> Phase1
    Phase1 -> Phase2 : [(slip_pred > 0.95*slip_max)]
    (junction 167) -> Phase2
    (junction 165) -> (junction 167)
    (junction 217) -> Phase1
    Phase2 -> Phase3 [order 2] : [(slip > 0.9*slip_max)]
    Phase3 -> Phase4 : [(slip < 0.9*slip_max)]
    Phase4 -> (junction 217) [order 1] : [(tq_cmd < tq_in)]
    (junction 220) -> (junction 217)
    Phase4 -> Phase5 [order 2] : [(sgn > 0)]
    Phase5 -> (junction 220) [order 1] : [(tq_cmd < tq_in)]
    Phase5 -> (junction 165) [order 2] : [(slip_pred > 0.9*slip_max)]
  state LSC_off
    entry,during:
    phase = 0;
  state ready
    phase = 0;
  LSC_On -> (junction 231) : [(coast_flag ~= 1)]
  (junction 231) -> ready
  (default) -> ready
  LSC_off -> LSC_On : [(sgn > 0)&&(slip > 0)&&(a_car < 0)]
  ready -> LSC_off : [(coast_flag == 1)]
  data: phase output; slip input; a_car input; coast_flag input; slip_pred input; slip_max input; tq_cmd input; tq_in input; sgn input; yaw_flag input

== stateflow chart SM_Tq_Ctrl/FR/Chart1 ==
  state LSC_On
    state Phase6
      entry,during:
      phase = 6;
    state Phase1
      entry,during:
      phase = 1;
    state Phase2
      entry,during:
      phase = 2;
    state Phase3
      entry,during:
      phase = 3;
    state Phase4
      entry,during:
      phase = 4;
    state Phase5
      entry,during:
      phase = 5;
    Phase6 -> (junction 225) [order 1] : [(yaw_flag == 1)]
    Phase6 -> (junction 235) [order 2] : [(slip > 0.85*slip_max)]
    (junction 225) -> Phase1
    (junction 235) -> (junction 167)
    Phase2 -> Phase6 [order 1] : [(slip_pred < 0.8*slip_max)]
    (default) -> Phase1
    Phase1 -> Phase2 : [(slip_pred > 0.95*slip_max)]
    (junction 167) -> Phase2
    (junction 165) -> (junction 167)
    (junction 217) -> Phase1
    Phase2 -> Phase3 [order 2] : [(slip > 0.9*slip_max)]
    Phase3 -> Phase4 : [(slip < 0.9*slip_max)]
    Phase4 -> (junction 217) [order 1] : [(tq_cmd < tq_in)]
    (junction 220) -> (junction 217)
    Phase4 -> Phase5 [order 2] : [(sgn > 0)]
    Phase5 -> (junction 220) [order 1] : [(tq_cmd < tq_in)]
    Phase5 -> (junction 165) [order 2] : [(slip_pred > 0.9*slip_max)]
  state LSC_off
    entry,during:
    phase = 0;
  state ready
    phase = 0;
  LSC_On -> (junction 231) : [(coast_flag ~= 1)]
  (junction 231) -> ready
  (default) -> ready
  LSC_off -> LSC_On : [(sgn > 0)&&(slip > 0)&&(a_car < 0)]
  ready -> LSC_off : [(coast_flag == 1)]
  data: phase output; slip input; a_car input; coast_flag input; slip_pred input; slip_max input; tq_cmd input; tq_in input; sgn input; yaw_flag input

== stateflow chart SM_Tq_Ctrl/FL/Chart1 ==
  state LSC_On
    state Phase6
      entry,during:
      phase = 6;
    state Phase1
      entry,during:
      phase = 1;
    state Phase2
      entry,during:
      phase = 2;
    state Phase3
      entry,during:
      phase = 3;
    state Phase4
      entry,during:
      phase = 4;
    state Phase5
      entry,during:
      phase = 5;
    Phase6 -> (junction 225) [order 1] : [(yaw_flag == 1)]
    Phase6 -> (junction 235) [order 2] : [(slip > 0.85*slip_max)]
    (junction 225) -> Phase1
    (junction 235) -> (junction 167)
    Phase2 -> Phase6 [order 1] : [(slip_pred < 0.8*slip_max)]
    (default) -> Phase1
    Phase1 -> Phase2 : [(slip_pred > 0.95*slip_max)]
    (junction 167) -> Phase2
    (junction 165) -> (junction 167)
    (junction 217) -> Phase1
    Phase2 -> Phase3 [order 2] : [(slip > 0.9*slip_max)]
    Phase3 -> Phase4 : [(slip < 0.9*slip_max)]
    Phase4 -> (junction 217) [order 1] : [(tq_cmd < tq_in)]
    (junction 220) -> (junction 217)
    Phase4 -> Phase5 [order 2] : [(sgn > 0)]
    Phase5 -> (junction 220) [order 1] : [(tq_cmd < tq_in)]
    Phase5 -> (junction 165) [order 2] : [(slip_pred > 0.9*slip_max)]
  state LSC_off
    entry,during:
    phase = 0;
  state ready
    phase = 0;
  LSC_On -> (junction 231) : [(coast_flag ~= 1)]
  (junction 231) -> ready
  (default) -> ready
  LSC_off -> LSC_On : [(sgn > 0)&&(slip > 0)&&(a_car < 0)]
  ready -> LSC_off : [(coast_flag == 1)]
  data: phase output; slip input; a_car input; coast_flag input; slip_pred input; slip_max input; tq_cmd input; tq_in input; sgn input; yaw_flag input

== stateflow chart SM_Tq_Ctrl/Coasting Torque Command/Slip Stateflow ==
  state Coasting
    state State0
      state = 0;
    state State1
      "No Slip"
      state = 1;
    state State2
      "Frnt Slip"
      state = 2;
    state State3
      "Rear Slip"
      state = 3;
    state State4
      "Both Slip"
      state = 4;
    (default) -> State0
    State0 -> State1 : [(ph_FL==1)&(ph_FR==1)&(ph_RL==1)&(ph_RR==1)]
    State1 -> State2 [order 1] : [(ph_FL~=1)|(ph_FR~=1)]
    State2 -> State1 [order 1] : [(ph_FL==1)&(ph_FR==1)]
    State3 -> State1 [order 1] : [(ph_RL==1)&(ph_RR==1)]
    State1 -> State3 [order 2] : [(ph_RL~=1)|(ph_RR~=1)]
    State4 -> State2 [order 1] : [(ph_RL==1)&(ph_RR==1)]
    State2 -> State4 [order 2] : [(ph_RL~=1)|(ph_RR~=1)]
    State3 -> State4 [order 2] : [(ph_FL~=1)|(ph_FR~=1)]
    State4 -> State3 [order 2] : [(ph_FL==1)&(ph_FR==1)]
  state drive
    state = 0;
  Coasting -> (junction 33) : [(coast_flag ~= 1)]
  (junction 33) -> drive
  (default) -> drive
  drive -> Coasting : [(coast_flag == 1)]
  data: coast_flag input; ph_FL input; ph_FR input; ph_RL input; ph_RR input; state output

== matlab function SM_Tq_Ctrl/Tire Force Estimation/MATLAB Function4 ==
  data: X input; w input; T input; X output; P output; P input; A input; r_e input; J input; M input; Ts input
function [X,P]  = fcn(X,w,T,P,A,r_e,J,M,Ts)

%X = [w_lf w_lr w_rf w_rr F_lf F_lr F_rf F_rr]
Q = diag([0.002 0.002 0.002 0.002 50 50 50 50]);

%Z = [w_lf w_lr w_rf w_rr ax]
Z = [w(1),w(2),w(3),w(4),A(1)]';
R = diag([0.002 0.002 0.002 0.002 0.02]);

U = [T(1) T(2) T(3) T(4)]';
G = [1/J 0 0 0;0 1/J 0 0;0 0 1/J 0;0 0 0 1/J;zeros(4,4)];

F = eye(8) + Ts*...
    [0 0 0 0 -r_e/J 0 0 0;
     0 0 0 0 0 -r_e/J 0 0;
     0 0 0 0 0 0 -r_e/J 0;
     0 0 0 0 0 0 0 -r_e/J;
     zeros(4,8)];

H = [eye(4) zeros(4,4);
     0 0 0 0 1/M 1/M 1/M 1/M];

Xm = F*X + G*U*Ts;
Pm = F*P*F'+Q;
K = Pm*H'/(H*Pm*H'+R);
X = Xm+K*(Z-H*Xm);
P = (eye(8)-K*H)*Pm;

% Fx = cos(St(1))*X(5)+X(6)+cos(St(2))*X(7)+X(8);
% 
% Crr = (Fx/M-A(1))/9.8;

== matlab function SM_Tq_Ctrl/FR/MATLAB Function ==
  data: slip input; slip_pred output; v_car input; a_car input; a_whl input; t_pred input; slip_sgn output
function [slip_pred,slip_sgn] = fcn(slip,v_car,a_car,a_whl,t_pred)

slip_sgn = (1-slip)*a_car-a_whl;
slip_pred = slip + 1/v_car*((1-slip)*a_car-a_whl)*t_pred;
% slip_pred = slip + 1/v_car*(-a_whl);

== matlab function SM_Tq_Ctrl/RR/MATLAB Function ==
  data: slip input; slip_pred output; v_car input; a_car input; a_whl input; t_pred input; slip_sgn output
function [slip_pred,slip_sgn] = fcn(slip,v_car,a_car,a_whl,t_pred)

slip_sgn = (1-slip)*a_car-a_whl;
slip_pred = slip + 1/v_car*((1-slip)*a_car-a_whl)*t_pred;
% slip_pred = slip + 1/v_car*(-a_whl);

== matlab function SM_Tq_Ctrl/RL/MATLAB Function ==
  data: slip input; slip_pred output; v_car input; a_car input; a_whl input; t_pred input; slip_sgn output
function [slip_pred,slip_sgn] = fcn(slip,v_car,a_car,a_whl,t_pred)

slip_sgn = (1-slip)*a_car-a_whl;
slip_pred = slip + 1/v_car*((1-slip)*a_car-a_whl)*t_pred;
% slip_pred = slip + 1/v_car*(-a_whl);

== matlab function SM_Tq_Ctrl/FL/MATLAB Function ==
  data: slip input; slip_pred output; v_car input; a_car input; a_whl input; t_pred input; slip_sgn output
function [slip_pred,slip_sgn] = fcn(slip,v_car,a_car,a_whl,t_pred)

slip_sgn = (1-slip)*a_car-a_whl;
slip_pred = slip + 1/v_car*((1-slip)*a_car-a_whl)*t_pred;
% slip_pred = slip + 1/v_car*(-a_whl);
